simulink model "neew2"  (R2016a)
settings: Solver=VariableStepAuto  StartTime=0.0  StopTime=10.0  RelTol=1e-3
libraries: nesl_utility x5, elec_lib x5, fl_lib x4, simulink x3
settings Model: Creator=ANSHUL  LastModifiedBy=ANSHUL

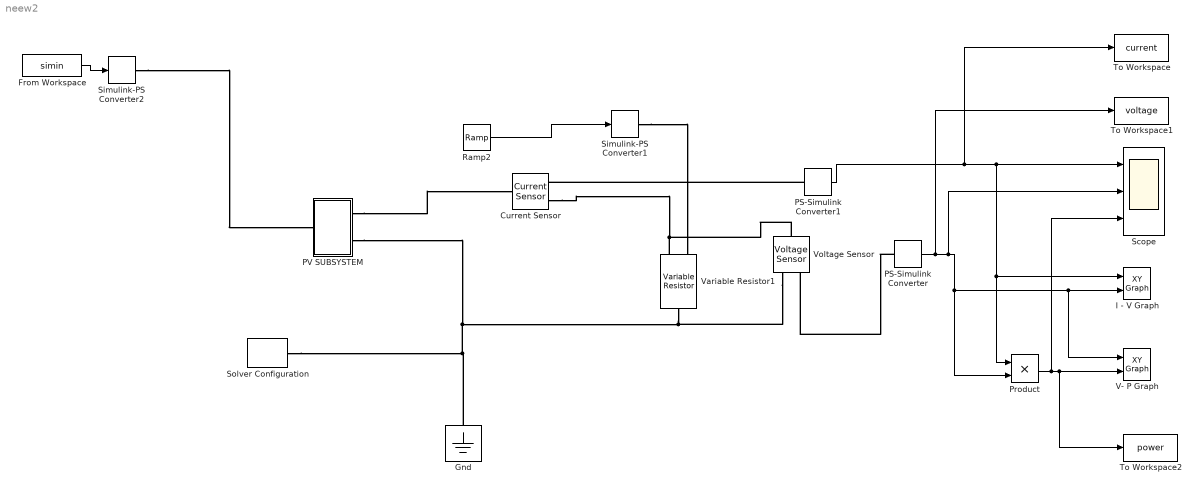
== system neew2 ==
  Current Sensor : fl_lib/Electrical/Electrical Sensors/Current Sensor
  From Workspace : FromWorkspace  VariableName=simin  SampleTime=10
  Gnd : fl_lib/Electrical/Electrical Elements/Electrical Reference
  I - V Graph : simulink/Sinks/XY Graph  xmin=0  xmax=100  ymin=0  ymax=2  st=0
  PS-Simulink Converter : nesl_utility/PS-Simulink Converter  PhysicalDomain=network_engine_domain  SubClassName=ps_output  LeftPortType=input  RightPortType=output  PseudoPeriodic=off  Frequencies=[]  Unit=1  AffineConversion=off
  PS-Simulink Converter1 : nesl_utility/PS-Simulink Converter  PhysicalDomain=network_engine_domain  SubClassName=ps_output  LeftPortType=input  RightPortType=output  PseudoPeriodic=off  Frequencies=[]  Unit=1  AffineConversion=off
  PV SUBSYSTEM : Subsystem
  Product : Product
  Ramp2 : simulink/Sources/Ramp  slope=1  start=0  X0=0
  Scope : Scope  NumInputPorts=3
  Simulink-PS Converter1 : nesl_utility/Simulink-PS Converter  PhysicalDomain=network_engine_domain  SubClassName=ps_input  LeftPortType=input  RightPortType=output  PseudoPeriodic=off  Frequencies=[]  NoiseDistribution=none  NoiseParameters=[]  Unit=1  AffineConversion=off  InputFiltering=off  SimscapeFilterOrder=1  InputFilterTimeConstant=0.001  UdotUserProvided=1
  Simulink-PS Converter2 : nesl_utility/Simulink-PS Converter  PhysicalDomain=network_engine_domain  SubClassName=ps_input  LeftPortType=input  RightPortType=output  PseudoPeriodic=off  Frequencies=[]  NoiseDistribution=none  NoiseParameters=[]  Unit=1  AffineConversion=off  InputFiltering=off  SimscapeFilterOrder=1  InputFilterTimeConstant=0.001  UdotUserProvided=1
  Solver Configuration : nesl_utility/Solver Configuration  PhysicalDomain=network_engine_domain  SubClassName=solver  LeftPortType=input  RightPortType=generic  Accelerate=off  Tones=[]  Harmonics=[]  SimulateNoise=off  Profile=off  UseLocalSampling=off  EnableSwitchedLinearOptims=on  FrequencyDomain=off  UseCCode=off  RelTol=0.001  AbsTol=1e-06  MinStep=1e-09  ToWorkspace=off  RevertToSquareIcSolve=off  NumHomotopyIterations=100  PhasorMode=off  PhasorModeNumHarmonics=1  OverrideAbsTol=off  DoDC=off  ResidualTolerance=1e-13  UseLocalSolver=on  LocalSolverChoice=NE_BACKWARD_EULER_ADVANCER  LocalSolverSampleTime=0.001  DoFixedCost=on  MaxNonlinIter=3  MaxModeIter=2  LinearAlgebra=Full  DelaysMemoryBudget=1024  AutomaticFiltering=on  FilteringTimeConstant=0.001
  To Workspace : ToWorkspace  VariableName=current  SampleTime=-1
  To Workspace1 : ToWorkspace  VariableName=voltage  SampleTime=-1
  To Workspace2 : ToWorkspace  VariableName=power  SampleTime=-1
  V- P Graph : simulink/Sinks/XY Graph  xmin=0  xmax=2  ymin=0  ymax=100  st=0
  Variable Resistor1 : fl_lib/Electrical/Electrical Elements/Variable Resistor  Rmin=0 Ohm  i_specify=off  i_priority=None  i=0 A  v_specify=off  v_priority=None  v=0 V
  Voltage Sensor : fl_lib/Electrical/Electrical Sensors/Voltage Sensor
  wires:
  Ramp2/1 -> Simulink-PS Converter1/1
  PS-Simulink Converter1/1 -> To Workspace/1, I - V Graph/1, Product/1, Scope/1
  PS-Simulink Converter/1 -> To Workspace1/1, Scope/2, V- P Graph/1, I - V Graph/2, Product/2
  Product/1 -> Scope/3, To Workspace2/1, V- P Graph/2
  From Workspace/1 -> Simulink-PS Converter2/1
  connections:
  Voltage Sensor/LConn1 -- Variable Resistor1/LConn2 -- Current Sensor/RConn2
  Gnd/LConn1 -- Solver Configuration/RConn1 -- PV SUBSYSTEM/RConn2 -- Variable Resistor1/RConn1 -- Voltage Sensor/RConn2
  PS-Simulink Converter1/LConn1 -- Current Sensor/RConn1
  PS-Simulink Converter/LConn1 -- Voltage Sensor/RConn1
  Simulink-PS Converter1/RConn1 -- Variable Resistor1/LConn1
  Simulink-PS Converter2/RConn1 -- PV SUBSYSTEM/LConn1
  PV SUBSYSTEM/RConn1 -- Current Sensor/LConn1

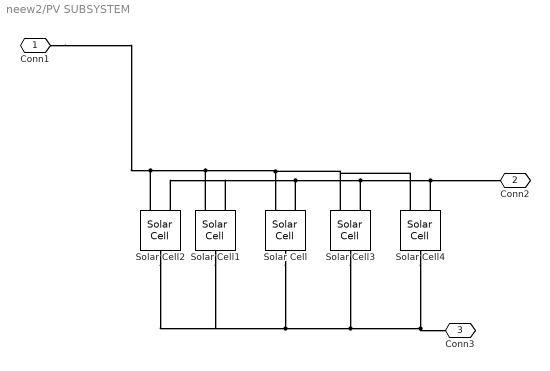
== system neew2/PV SUBSYSTEM ==
  Solar Cell{,1..4} (5 alike) : elec_lib/Sources/Solar Cell  prm=1  Isc=7.34 A  Voc=1.2 V  Is=1e-6 A  Is2=0 A  Iph=7.34 A  Ir0=1000 W/m^2  ec=1  N2=2  Rs=0 Ohm  Rp=Inf Ohm  N_series=1  TIPH1=1 1/K  EG=1.11 eV  TXIS1=3  TXIS2=3  TRS1=0  TRP1=0  Tmeas=25 degC  TFIXED=25 degC  thermal_mass=100 J/K  initial_temperature=25 degC
  Conn1 : PMIOPort  Port=1  Side=Left
  Conn2 : PMIOPort  Port=2  Side=Right
  Conn3 : PMIOPort  Port=3  Side=Right
  connections:
  Solar Cell2/LConn1 -- Conn1/RConn1 -- Solar Cell1/LConn1 -- Solar Cell4/LConn1 -- Solar Cell3/LConn1 -- Solar Cell/LConn1
  Solar Cell/LConn2 -- Solar Cell2/LConn2 -- Solar Cell1/LConn2 -- Solar Cell3/LConn2 -- Conn2/RConn1 -- Solar Cell4/LConn2
  Solar Cell3/RConn1 -- Conn3/RConn1 -- Solar Cell4/RConn1 -- Solar Cell1/RConn1 -- Solar Cell2/RConn1 -- Solar Cell/RConn1
